simulink model "test_serial_com_PC"  (R2018a)
settings: Solver=FixedStepDiscrete  StartTime=0.0  StopTime=inf  FixedStep=1/100  RelTol=1e-3
undefined symbols (not defined in the file): serial
libraries: instrumentlib x3, etargetslib x2, sldrtlib x1, aerolibanimutils x1
settings Model: Creator=Myschik  LastModifiedBy=hiepp

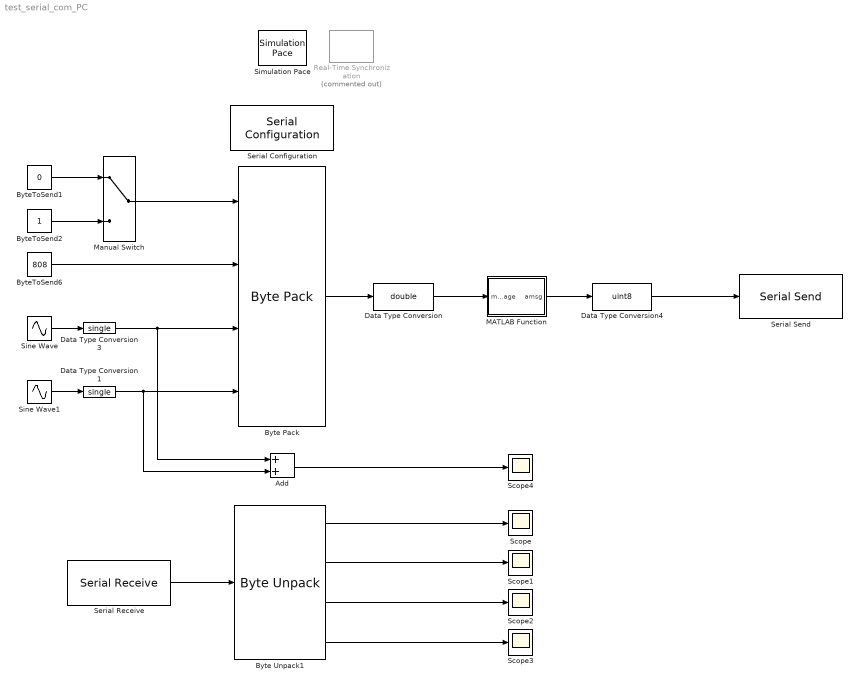
== system test_serial_com_PC ==
  Add : Sum
  Byte Pack : etargetslib/Byte Pack  datatypes={'single','single','single','single'}  byteAlign=1
  Byte Unpack1 : etargetslib/Byte Unpack  dimensions={[1],[1],[1],[1]}  datatypes={'single','single','single','single'}  byteAlign=1
  ByteToSend1 : Constant  Value=0  OutDataTypeStr=single  SampleTime=-1
  ByteToSend2 : Constant  OutDataTypeStr=single  SampleTime=-1
  ByteToSend6 : Constant  Value=808  OutDataTypeStr=single  SampleTime=-1
  Data Type Conversion : DataTypeConversion  OutDataTypeStr=double
  Data Type Conversion1 : DataTypeConversion  OutDataTypeStr=single
  Data Type Conversion3 : DataTypeConversion  OutDataTypeStr=single
  Data Type Conversion4 : DataTypeConversion  OutDataTypeStr=uint8
  MATLAB Function : MATLAB Function  TreatAsAtomicUnit=on
  Manual Switch : ManualSwitch
  Real-Time Synchronization : sldrtlib/Real-Time Synchronization  Commented=on  SampleTime=0.1  MaxMissedTicks=10  ShowMissedTicks=off  YieldWhenWaiting=off
  Scope{,1..4} (5 alike) : Scope
  Serial Configuration : instrumentlib/Serial Configuration  Priority=-200000  ComPortMenu=COM4  ComPort=COM4  ObjConstructor=serial('COM4');  BaudRate=115200  DataBits=8  Parity=none  StopBits=1  FlowControl=none  Timeout=10  ByteOrder=LittleEndian
  Serial Receive : instrumentlib/Serial Receive  ComPortMenu=COM4  ComPort=COM4  ObjConstructor=serial('COM4');  Terminator=<none>  DataSize=16  DataType=uint8  EnableBlockingMode=on  ActionDataUnavailable=Output last received value  CustomValue=0  SampleTime=0.01
  Serial Send : instrumentlib/Serial Send  ComPortMenu=COM4  ComPort=COM4  ObjConstructor=serial('COM4');  Header=\nn  Terminator=<none>  EnableBlockingMode=off
  Simulation Pace : aerolibanimutils/Simulation Pace  SimulationPace=1  SleepMode=MATLAB Thread  OutputPaceError=off  SampleTime=-1
  Sine Wave : Sin  Amplitude=10  SampleTime=0
  Sine Wave1 : Sin  Amplitude=10  Frequency=2  Phase=45*pi/180  SampleTime=0
  wires:
  Sine Wave/1 -> Data Type Conversion3/1
  Sine Wave1/1 -> Data Type Conversion1/1
  Data Type Conversion3/1 -> Add/1, Byte Pack/3
  ByteToSend6/1 -> Byte Pack/2
  MATLAB Function/1(amsg) -> Data Type Conversion4/1
  Byte Pack/1 -> Data Type Conversion/1
  Data Type Conversion/1 -> MATLAB Function/1(message)
  Data Type Conversion4/1 -> Serial Send/1
  Data Type Conversion1/1 -> Add/2, Byte Pack/4
  Serial Receive/1 -> Byte Unpack1/1
  Add/1 -> Scope4/1
  ByteToSend1/1 -> Manual Switch/1
  ByteToSend2/1 -> Manual Switch/2
  Manual Switch/1 -> Byte Pack/1
  Byte Unpack1/4 -> Scope3/1
  Byte Unpack1/3 -> Scope2/1
  Byte Unpack1/2 -> Scope1/1
  Byte Unpack1/1 -> Scope/1

== matlab function test_serial_com_PC/MATLAB Function ==
  data: message input; amsg output
function amsg = crc_Calc(message)
% Appends the crc (Low byte, high byte) to message for modbus
% communication. Message is an array of bytes. Developed for (but not
% limmited to) use with a watlow 96 controller.
amsg = zeros(18,1);
N = length(message);
Crc_ui16LookupTable=[0,4129,8258,12387,16516,20645,24774,28903,33032,37161,41290,45419,49548,...
    53677,57806,61935,4657,528,12915,8786,21173,17044,29431,25302,37689,33560,45947,41818,54205,...
    50076,62463,58334,9314,13379,1056,5121,25830,29895,17572,21637,42346,46411,34088,38153,58862,...
    62927,50604,54669,13907,9842,5649,1584,30423,26358,22165,18100,46939,42874,38681,34616,63455,...
    59390,55197,51132,18628,22757,26758,30887,2112,6241,10242,14371,51660,55789,59790,63919,35144,...
    39273,43274,47403,23285,19156,31415,27286,6769,2640,14899,10770,56317,52188,64447,60318,39801,...
    35672,47931,43802,27814,31879,19684,23749,11298,15363,3168,7233,60846,64911,52716,56781,44330,...
    48395,36200,40265,32407,28342,24277,20212,15891,11826,7761,3696,65439,61374,57309,53244,48923,...
    44858,40793,36728,37256,33193,45514,41451,53516,49453,61774,57711,4224,161,12482,8419,20484,...
    16421,28742,24679,33721,37784,41979,46042,49981,54044,58239,62302,689,4752,8947,13010,16949,...
    21012,25207,29270,46570,42443,38312,34185,62830,58703,54572,50445,13538,9411,5280,1153,29798,...
    25671,21540,17413,42971,47098,34713,38840,59231,63358,50973,55100,9939,14066,1681,5808,26199,...
    30326,17941,22068,55628,51565,63758,59695,39368,35305,47498,43435,22596,18533,30726,26663,6336,...
    2273,14466,10403,52093,56156,60223,64286,35833,39896,43963,48026,19061,23124,27191,31254,2801,6864,...
    10931,14994,64814,60687,56684,52557,48554,44427,40424,36297,31782,27655,23652,19525,15522,11395,...
    7392,3265,61215,65342,53085,57212,44955,49082,36825,40952,28183,32310,20053,24180,11923,16050,3793,7920];

data=[message]; % ~ string '1 2 3 4 5 6 7 8 9'

ui16RetCRC16 = hex2dec('0000');
for I=1:length(data)
    ui8LookupTableIndex = bitxor(data(I),uint8(bitshift(ui16RetCRC16,-8)));
    ui16RetCRC16 = bitxor(Crc_ui16LookupTable(double(ui8LookupTableIndex)+1),mod(bitshift(ui16RetCRC16,8),65536));
end

lowByte = bitand(ui16RetCRC16,hex2dec('ff'));
highByte = bitshift(bitand(ui16RetCRC16,hex2dec('ff00')),-8);

% 
% lowByte = bitand(crc,hex2dec('ff'));
% highByte = bitshift(bitand(crc,hex2dec('ff00')),-8);

amsg(1:N) = message;
amsg(N+1) = lowByte;
amsg(N+2) = highByte;
